simulink model "ex_lateral_kinematic"  (R2026a)
settings: Solver=VariableStepAuto
libraries: aerolibconvert2 x2
settings Model: Creator=doyeop  LastModifiedBy=doyeop

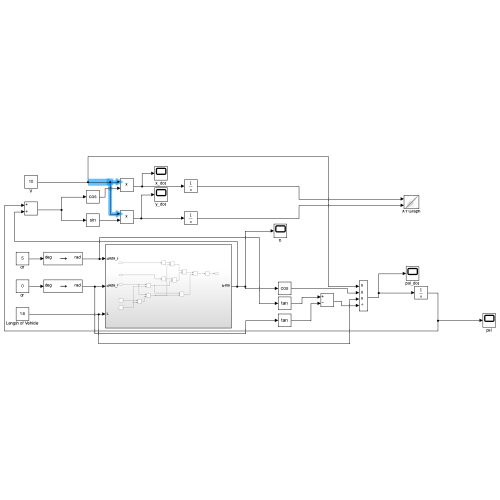
[thumbnail: Simulink's stored preview of the top-level diagram]
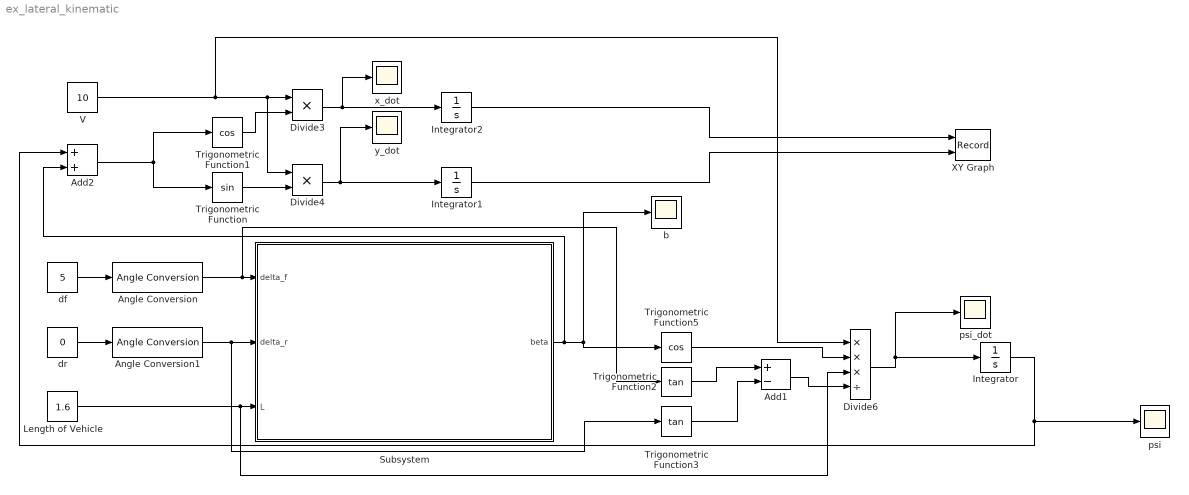
== system ex_lateral_kinematic ==
  Add1 : Sum  Inputs=+-
  Add2 : Sum
  Angle Conversion : aerolibconvert2/Angle Conversion  IU=deg  OU=rad
  Angle Conversion1 : aerolibconvert2/Angle Conversion  IU=deg  OU=rad
  Divide3 : Product  Inputs=**
  Divide4 : Product  Inputs=**
  Divide6 : Product  Inputs=***/
  Integrator : Integrator
  Integrator1 : Integrator
  Integrator2 : Integrator
  Length of Vehicle : Constant  Value=1.6
  Subsystem : Subsystem
  Trigonometric Function : Trigonometry
  Trigonometric Function1 : Trigonometry  Operator=cos
  Trigonometric Function2 : Trigonometry  Operator=tan
  Trigonometric Function3 : Trigonometry  Operator=tan
  Trigonometric Function5 : Trigonometry  Operator=cos
  V : Constant  Value=10  SampleTime=-1
  XY Graph : Record  NumPorts=2.0  FileSettingsInternal="{\"entries\":[{\"content\":{\"excelSettings\":{\"content\":{},\"type\":\"Streamout.ExcelSettings\"},\"parquetSettings\":{\"content\":{},\"type\":\"Streamout.ParquetSettings\"}},\"type\":\"Streamout.FileSettingStorage\",\"uuid\":\"\"}],\"packageUris\":[\"http:\\/\\/schema.mathworks.com\\/mf0\\/streamout_blocks\\/R2020a\"],\"version\":\"1.0\"}"  FrameSettings=[0, 0]  Layout=[1 1]  SignalsInternal="{\"entries\":[{\"content\":{\"signals\":[{\"content\":{\"blockPath\":[],\"dimensions\":[1],\"domain\":\"\",\"lineColor\":\"#a2142f\",\"plots\":[ 1 ],\"port\":1,\"sid\":[\"\"],\"signalID\":1,\"signalName\":\"Integrator2\"},\"type\":\"RecordBlkView.Signal\",\"uuid\":\"\"},{\"content\":{\"blockPath\":[],\"dimensions\":[1],\"domain\":\"\",\"lineColor\":\"#139fff\",\"plots\":[ 1 ],\"port\":2,\"sid\":[\"\"],\"signalID\":2,\"signalName\":\"Integrator1\"},\"type\":\"RecordBlkView.Signal\",\"uuid\":\"\"}]},\"type\":\"RecordBlkView.InputSignals\",\"uuid\":\"\"}],\"packageUris\":[\"http:\\/\\/schema.mathworks.com\\/mf0\\/streamout_blocks\\/R2020a\"],\"version\":\"1.0\"}"  VisualizationBindings="{\"xyplotplugin\":{\"info\":[{\"series\":[{\"bindingParametersList\":[{\"parameter\":\"X-Axis\",\"signalID\":1,\"signalName\":\"Integrator2\"},{\"parameter\":\"Y-Axis\",\"signalID\":2,\"signalName\":\"Integrator1\"}],\"seriesID\":0}],\"subplotID\":1}]}}"  CompatibilityTag=XY
  b : Scope
      settings: ActiveDisplayYMinimum=-1  ActiveDisplayYMaximum=1
  df : Constant  Value=5  SampleTime=-1
  dr : Constant  Value=0  SampleTime=-1
  psi : Scope
      settings: ActiveDisplayYMinimum=-13079.866508029954  ActiveDisplayYMaximum=117718.79857226962  DataLoggingVariableName=ScopeData4
  psi_dot : Scope
      settings: ActiveDisplayYMinimum=82.629389029164827  ActiveDisplayYMaximum=282.62938902916483
  x_dot : Scope
      settings: ActiveDisplayYMinimum=-1  ActiveDisplayYMaximum=1  DataLoggingVariableName=ScopeData2
  y_dot : Scope
      settings: ActiveDisplayYMinimum=-1  ActiveDisplayYMaximum=1  DataLoggingVariableName=ScopeData3
  wires:
  V/1 -> Divide3/1, Divide4/1, Divide6/1
  Trigonometric Function1/1 -> Divide3/2
  Trigonometric Function/1 -> Divide4/2
  Trigonometric Function5/1 -> Divide6/2
  Subsystem/1(beta) -> Add2/2, b/1, Trigonometric Function5/1
  df/1 -> Angle Conversion/1
  dr/1 -> Angle Conversion1/1
  Length of Vehicle/1 -> Divide6/3, Subsystem/3(L)
  Trigonometric Function2/1 -> Add1/1
  Trigonometric Function3/1 -> Add1/2
  Add1/1 -> Divide6/4
  Divide6/1 -> Integrator/1, psi_dot/1
  Add2/1 -> Trigonometric Function1/1, Trigonometric Function/1
  Divide3/1 -> Integrator2/1, x_dot/1
  Divide4/1 -> Integrator1/1, y_dot/1
  Integrator2/1 -> XY Graph/1
  Integrator1/1 -> XY Graph/2
  Angle Conversion/1 -> Trigonometric Function2/1, Subsystem/1(delta_f)
  Angle Conversion1/1 -> Subsystem/2(delta_r), Trigonometric Function3/1
  Integrator/1 -> psi/1, Add2/1

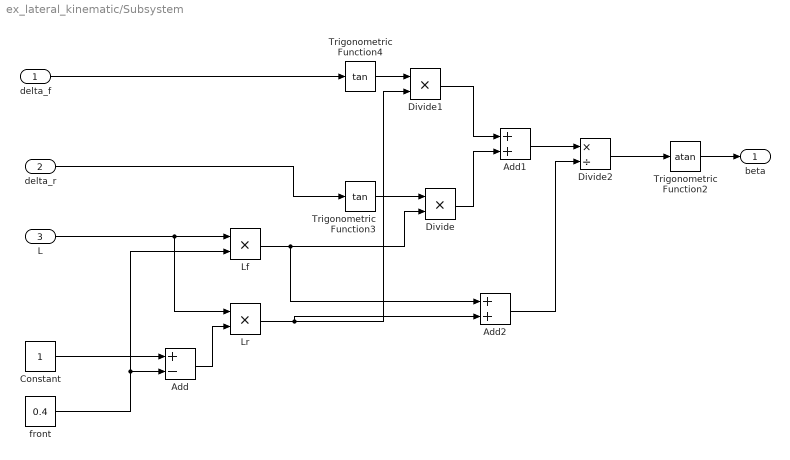
== system ex_lateral_kinematic/Subsystem ==
  delta_f : Inport
  delta_r : Inport  Port=2
  L : Inport  Port=3
  Add : Sum  Inputs=+-
  Add1 : Sum
  Add2 : Sum
  Constant : Constant  SampleTime=-1
  Divide : Product  Inputs=**
  Divide1 : Product  Inputs=**
  Divide2 : Product  Inputs=*/
  Lf : Product
  Lr : Product
  Trigonometric Function2 : Trigonometry  Operator=atan
  Trigonometric Function3 : Trigonometry  Operator=tan
  Trigonometric Function4 : Trigonometry  Operator=tan
  front : Constant  Value=0.4  SampleTime=-1
  beta : Outport
  wires:
  Trigonometric Function4/1 -> Divide1/1
  Lf/1 -> Add2/1, Divide/2
  Add1/1 -> Divide2/1
  Trigonometric Function2/1 -> beta/1
  front/1 -> Lf/2, Add/2
  Constant/1 -> Add/1
  delta_r/1 -> Trigonometric Function3/1
  Divide/1 -> Add1/2
  Trigonometric Function3/1 -> Divide/1
  Divide2/1 -> Trigonometric Function2/1
  L/1 -> Lr/1, Lf/1
  delta_f/1 -> Trigonometric Function4/1
  Lr/1 -> Add2/2, Divide1/2
  Add2/1 -> Divide2/2
  Divide1/1 -> Add1/1
  Add/1 -> Lr/2
